simulink model "LF_AC29bus_HVDCdemo_V2_1"  (R2019b)
settings: Solver=FixedStepDiscrete  StartTime=0.0  StopTime=fix(6/Ts)*Ts  FixedStep=Ts  RelTol=1e-3
InitFcn:
  | Ts_avg=150e-6;
  | Ts=50e-6;
  | 
  | %Tc_stab = 1/60/5;
  | %Tc_stab = 2/60;
  | Tc_stab = Ts;
  | 
  | 
  | Ts_avg=150e-6;
  | 
  | Ts=50e-6;
  | 
  | % Rectifier AC side :
  | VLL_nom_R = 735e3; % V
  | Fnom_R = 60;           % Hz
  | 
  | % Inverter AC side :
  | VLL_nom_I = 735e3; % V
  | Fnom_I = 60;           % Hz
  | 
  | % DC :
  | Vdc_nom = 500e3;   % V
  | Idc_nom  = 2000;     % A
undefined symbols (not defined in the file): D1, D11, Delta, test_alpha
libraries: powerlib x223, powerlib_meascontrol x57, simulink x22, sps_avr x7
(part 9 of 10)

== system LF_AC29bus_HVDCdemo_V2_1/HVDC_network_avg/Inverter Control and Protection (Average model)/Inverter Protections/Commutation Failure Prevention Control (CFPREV)/CFPREV ==
  note: Ref. "A Novel Method to Mitigate Commutation Failures in HVDC Systems,"
      | Lidong Zhang, Lars Dofnas ABB Utilities Power System Technology,
      | Proceedings PowerCon 2002, Volume: 1 , 13-17 Oct. 2002,  Page(s): 51-56 vol.1
  note: Silvano Casoria
      | Power System Laboratory, IREQ
      | Hydro-Quebec
  note: Commutation failure Prevention Control (CFPREV)
  note: Fast initialisation
      | for simulation
  Uabc (pu) : Inport
  Enable (Held) : EnablePort  PropagateVarSize=During execution
  AB_LEVEL : Constant  Value=ab_level
  ALPFA_BETA_SUM : Fcn  Expr=sqrt(u[1]^2+u[2]^2)
  ALPFA_BETA_SUM1 : Fcn  Expr=abs(u[3]) * 3
  C : Constant  Value=filt_tc
  C1 : Constant  Value=1/(fn)
  Discrete Shift Register 1 (T_periode) : powerlib_meascontrol/Additional Components/Discrete Shift Register  NSamples=fix(T_periode/Ts)  InitialValue=0  Ts=Ts
      settings: SourceProductName=Simscape Electrical  SourceProductBaseCode=PS
  Discrete Shift Register 2 (T_periode) : powerlib_meascontrol/Additional Components/Discrete Shift Register  NSamples=fix(T_periode/Ts)  InitialValue=0  Ts=Ts
      settings: SourceProductName=Simscape Electrical  SourceProductBaseCode=PS
  First-Order Filter (T=0.03) : powerlib_meascontrol/Filters/First-Order Filter  FilterType=Lowpass  Tc=0.03  Ts=Ts  Initialize=off  Vac_Init=[0, 0, Fnom_I]  Vdc_Init=0  PlotResponse=off  FreqRange="[0,  200,  1]"
      settings: SourceProductName=Simscape Electrical
  Gain : Gain  Gain=ab_gain  SaturateOnIntegerOverflow=on  OutDataTypeStr=Inherit: Same as input  ParamDataTypeStr=Inherit: Same as input
  "Gain  " : Gain  Gain=z_gain  SaturateOnIntegerOverflow=on  OutDataTypeStr=Inherit: Same as input  ParamDataTypeStr=Inherit: Same as input
  Ground : Ground
  Low Pass (IC = filt_ic) : Subsystem  mask(Low Pass Filter With Reset (discrete: Zoh method, Forward Euler)){ic=filt_ic, dt=Ts}
      mask prompts: ic "Initial condition:"; dt "Sample time (s)"
      mask help:
      | The output will be reset to the input value (Time constant = 0)  during the input (2) is True. The Time constant (T) is defined by
      | input (3).
      mask Display:
      | plot(0,0,100,100,[90,80,70,60,50,40,29,20,10],[60,55,52,55,60,65,67,65,60],[89,80,71,60,50,40,30,20,10],[40,35,32,35,40,45,47,45,40],[56,44],[70,50]);
      | disp('\n\nD')
  Max: 1 pu Min = 0 : Saturate  UpperLimit=1.0  LowerLimit=0
  MinMax1 : MinMax  Function=max  SaturateOnIntegerOverflow=on  InputSameDT=on
  MinMax2 : MinMax  Function=max  SaturateOnIntegerOverflow=on  InputSameDT=on
  MinMax3 : MinMax  Function=max  Inputs=2  SaturateOnIntegerOverflow=on  InputSameDT=on
  MinMax4 : MinMax  Function=max  Inputs=2  SaturateOnIntegerOverflow=on  InputSameDT=on
  Relational Operator : RelationalOperator  Operator=>  RndMeth=Nearest
  Relational Operator1 : RelationalOperator  Operator=>  RndMeth=Nearest
  Sum : Sum  Inputs=+-  SaturateOnIntegerOverflow=on
  Switch : Switch  Criteria=u2 > Threshold  SaturateOnIntegerOverflow=on
  Switch1 : Switch  Criteria=u2 > Threshold  SaturateOnIntegerOverflow=on
  Switch2 : Switch  Criteria=u2 > Threshold  SaturateOnIntegerOverflow=on
  T_ss : Step  Time=T_ss  Before=1  After=0  SampleTime=0
  ZERO : Constant  Value=0
  ZERO1 : Constant  Value=0
  Z_LEVEL : Constant  Value=z_level
  abc to Alpha-Beta-Zero : powerlib_meascontrol/Transformations/abc to Alpha-Beta-Zero
      settings: SourceProductName=Simscape Electrical
  AMIN_CFPREV (deg) : Outport
  wires:
  MinMax4/1 -> AMIN_CFPREV (deg)/1
  MinMax3/1 -> First-Order Filter (T=0.03)/1, MinMax4/2
  ALPFA_BETA_SUM/1 -> Low Pass (IC = filt_ic)/1(In), Sum/2
  Sum/1 -> Discrete Shift Register 2 (T_periode)/1, Relational Operator/1
  AB_LEVEL/1 -> Relational Operator/2
  Relational Operator/1 -> Switch/2  "AB_DET"
  Discrete Shift Register 2 (T_periode)/1 -> MinMax1/1
  MinMax1/1 -> Gain/1
  Gain/1 -> Switch/1  "AB_AMIN"
  ZERO/1 -> Switch/3
  ALPFA_BETA_SUM1/1 -> Discrete Shift Register 1 (T_periode)/1, Relational Operator1/1  "Z_DIFF"
  Z_LEVEL/1 -> Relational Operator1/2
  Discrete Shift Register 1 (T_periode)/1 -> MinMax2/1
  MinMax2/1 -> Max: 1 pu Min = 0/1
  Max: 1 pu Min = 0/1 -> "Gain  "/1
  Relational Operator1/1 -> Switch1/2  "Z_DET"
  "Gain  "/1 -> Switch1/1  "Z_AMIN"
  ZERO1/1 -> Switch1/3
  Switch/1 -> MinMax3/1  "AB MIN"
  Switch1/1 -> MinMax3/2  "Z MIN"
  abc to Alpha-Beta-Zero/1 -> ALPFA_BETA_SUM/1, ALPFA_BETA_SUM1/1
  Uabc (pu)/1 -> abc to Alpha-Beta-Zero/1
  Low Pass (IC = filt_ic)/1(Out) -> Sum/1
  Switch2/1 -> Low Pass (IC = filt_ic)/3(T)
  C/1 -> Switch2/3
  T_ss/1 -> Switch2/2
  C1/1 -> Switch2/1
  Ground/1 -> Low Pass (IC = filt_ic)/2(R)
  First-Order Filter (T=0.03)/1 -> MinMax4/1

== system LF_AC29bus_HVDCdemo_V2_1/HVDC_network_avg/Inverter Control and Protection (Average model)/Inverter Protections/Low  AC Voltage Detection (LACVD)/LACVD ==
  note: Low AC Voltage Detection
  Uac (pu) : Inport
  Enable (Held) : EnablePort  PropagateVarSize=During execution
  Off Delay : powerlib_meascontrol/Logic/On Delay  DelayType=Off delay  delay=0.009  ic=0  Ts=Ts
      settings: SourceProductName=Simscape Electrical
  "On Delay 1 " : powerlib_meascontrol/Logic/On Delay  DelayType=On delay  delay=0.001  ic=0  Ts=Ts
      settings: SourceProductName=Simscape Electrical
  On Delay 2 : powerlib_meascontrol/Logic/On Delay  DelayType=On delay  delay=0.014  ic=0  Ts=Ts
      settings: SourceProductName=Simscape Electrical
  REF_1 (pu) : Constant  Value=Ref_1
  Relational Operator1 : RelationalOperator  Operator=<=  RndMeth=Nearest  InputSameDT=on
  Low_AC_Voltage : Outport
  wires:
  REF_1 (pu)/1 -> Relational Operator1/2
  Uac (pu)/1 -> Relational Operator1/1
  "On Delay 1 "/1 -> Off Delay/1
  Off Delay/1 -> On Delay 2/1
  Relational Operator1/1 -> "On Delay 1 "/1
  On Delay 2/1 -> Low_AC_Voltage/1

== system LF_AC29bus_HVDCdemo_V2_1/HVDC_network_avg/Rectifier Average model/HVDC_CONV_AVG/Average Model Computation/Iabc_calc ==
  note: Iabc_calc
  note: Iabc Calculation
  I_dq : Inport
  theta : Inport  Port=2
  Constant : Constant  Value=0
  Mux : Mux  Inputs=[2 1]
  dq0 to abc : powerlib_meascontrol/Transformations/dq0 to abc  Alignment=90 degrees behind phase A axis
      settings: SourceProductName=Simscape Electrical
  rms->peak : Gain  Gain=sqrt(2)
  Iabc : Outport
  wires:
  Mux/1 -> dq0 to abc/1
  dq0 to abc/1 -> Iabc/1
  theta/1 -> dq0 to abc/2
  Constant/1 -> Mux/2
  I_dq/1 -> rms->peak/1
  rms->peak/1 -> Mux/1

== system LF_AC29bus_HVDCdemo_V2_1/HVDC_network_avg/Rectifier Average model/HVDC_CONV_AVG/Average Model Computation/Ud_calc_dyn ==
  note: Derivative
  note: (2 - mu_deg/120) * Lc
  note: dId/dt
  note: Band pass limitation
  note: Output limitation
  note: Ud_calc_dyn
  note: Inductive voltage drop calculation due to current variation
  note: Mean commutation inductance,
      | a function of the commutation interval
  Id : Inport
  mu_deg : Inport  Port=2
  Ud_tmp : Inport  Port=3
  Add : Sum  Inputs=-+
  Difference : Subsystem  mask(Difference){ICPrevInput=0, OutMin=[], OutMax=[], OutDataTypeStr=Inherit: Inherit via internal rule, OutputDataTypeScalingMode=Inherit via internal rule, OutDataType=fixdt(1, 16), OutScaling=2^-10, LockScale=off, RndMeth=Floor, DoSatur=off}
      mask prompts: ICPrevInput "Initial condition for previous input:"; OutMin "Output minimum:"; OutMax "Output maximum:"; OutDataTypeStr "Output data type:"; OutputDataTypeScalingMode "Output data type mode:"; OutDataType "Output data type (e.g. fixdt(1, 16), fixdt('single')):"; OutScaling "Output scaling (Slope, e.g. 2^-9 or [Slope Bias], e.g. [1.25 3]):"; LockScale "Lock output data type setting against changes by the fixed-point tools"; RndMeth "Integer rounding mode:"; DoSatur "Saturate to max or min when overflows occur"
      mask help: Output the current input value minus the previous input value.
      mask init:
      | blkH = gcbh;
      | blkName = getfullname(blkH);
      | 
      | set_param([blkName,'/Diff'], ...
      |     'RndMeth',RndMeth, ...
      | 	'DoSatur',DoSatur);
      mask Callback OutDataTypeStr: fixptdialog(gcbh)
      mask TypeOptions OutputDataTypeScalingMode: double | single | int8 | uint8 | int16 | uint16 | int32 | uint32 | Specify via dialog | Inherit via internal rule | Inherit via back propagation
      mask Callback OutputDataTypeScalingMode: fixptdialog(gcbh)
      mask Callback OutDataType: fixptdialog(gcbh)
      mask TypeOptions RndMeth: Ceiling | Convergent | Floor | Nearest | Round | Simplest | Zero
      mask Display: dpoly([1 -1],[1 0],'z')
  Difference (IC: Ts) : Subsystem  mask(Difference){ICPrevInput=Ts, OutMin=[], OutMax=[], OutDataTypeStr=Inherit: Inherit via internal rule, OutputDataTypeScalingMode=Inherit via internal rule, OutDataType=fixdt(1, 16), OutScaling=2^-10, LockScale=off, RndMeth=Floor, DoSatur=off}
      mask prompts: ICPrevInput "Initial condition for previous input:"; OutMin "Output minimum:"; OutMax "Output maximum:"; OutDataTypeStr "Output data type:"; OutputDataTypeScalingMode "Output data type mode:"; OutDataType "Output data type (e.g. fixdt(1, 16), fixdt('single')):"; OutScaling "Output scaling (Slope, e.g. 2^-9 or [Slope Bias], e.g. [1.25 3]):"; LockScale "Lock output data type setting against changes by the fixed-point tools"; RndMeth "Integer rounding mode:"; DoSatur "Saturate to max or min when overflows occur"
      mask help: Output the current input value minus the previous input value.
      mask init:
      | blkH = gcbh;
      | blkName = getfullname(blkH);
      | 
      | set_param([blkName,'/Diff'], ...
      |     'RndMeth',RndMeth, ...
      | 	'DoSatur',DoSatur);
      mask Callback OutDataTypeStr: fixptdialog(gcbh)
      mask TypeOptions OutputDataTypeScalingMode: double | single | int8 | uint8 | int16 | uint16 | int32 | uint32 | Specify via dialog | Inherit via internal rule | Inherit via back propagation
      mask Callback OutputDataTypeScalingMode: fixptdialog(gcbh)
      mask Callback OutDataType: fixptdialog(gcbh)
      mask TypeOptions RndMeth: Ceiling | Convergent | Floor | Nearest | Round | Simplest | Zero
      mask Display: dpoly([1 -1],[1 0],'z')
  Digital Clock : DigitalClock  SampleTime=Ts
  Divide : Product  Inputs=*/
  Fcn : Fcn  Expr=(2 - u(1)/120)*Lc
  First-Order Filter (T=0.0005) : powerlib_meascontrol/Filters/First-Order Filter  FilterType=Lowpass  Tc=0.0005  Ts=Ts  Initialize=off  Vac_Init=[0, 0, 60]  Vdc_Init=0  PlotResponse=off  FreqRange="[0,  200,  1]"
      settings: SourceProductName=Simscape Electrical
  Max:10*Usec Min:-10*Usec : Saturate  UpperLimit=10*Usec  LowerLimit=-10*Usec
  Product : Product  RndMeth=Zero
  Ud : Outport
  wires:
  Product/1 -> Add/1
  Difference (IC: Ts)/1(Y) -> Divide/2
  Digital Clock/1 -> Difference (IC: Ts)/1(U)
  Id/1 -> Difference/1(U)
  Divide/1 -> First-Order Filter (T=0.0005)/1
  Difference/1(Y) -> Divide/1
  Fcn/1 -> Product/1  "mean_Lc"
  mu_deg/1 -> Fcn/1
  Add/1 -> Max:10*Usec Min:-10*Usec/1
  Ud_tmp/1 -> Add/2
  First-Order Filter (T=0.0005)/1 -> Product/2
  Max:10*Usec Min:-10*Usec/1 -> Ud/1

== system LF_AC29bus_HVDCdemo_V2_1/HVDC_network_avg/Rectifier Average model/HVDC_CONV_AVG/Average Model Computation/Udi0_calc ==
  note: Np/Ns (pu)
  note: Udi0_calc
  note: 3*sqrt(2)/pi * Usec_nom
  note: Udio Calculation
  Uabc : Inport
  Tap_pu : Inport  Port=2
  Avoid zero : Saturate  UpperLimit=inf  LowerLimit=eps
  "Avoid zero " : Saturate  UpperLimit=inf  LowerLimit=eps
  Divide3 : Product  Inputs=*/
  PLL (3ph) : powerlib_meascontrol/PLL/PLL (3ph)  Fmin=0.75 * fn  Par_Init="[0  fn]"  ParK=[60 1400 0]  TcD=Ts  MaxRateChangeFreq=12  FilterCutOffFreq=25  Ts=Ts  AGC=off
      settings: SourceProductName=Simscape Electrical
  Positive-Sequence (PLL-Driven) : powerlib_meascontrol/Measurements/Positive-Sequence (PLL-Driven)  Finit=fn  Fmin=45  InInit=[1, 0]  Ts=Ts
      settings: SourceProductName=Simscape Electrical  SourceProductBaseCode=PS
  Terminator1 : Terminator
  V->pu : Gain  Gain=1/(Uprim/sqrt(1.5))
  V->pu1 : Gain  Gain=2*pi
  delay compensation : Subsystem
  pu->Udio_V : Gain  Gain=(3*sqrt(2)/pi) * Usec
  Udi0 : Outport
  w : Outport  Port=2
  theta : Outport  Port=3
  wires:
  PLL (3ph)/2 -> delay compensation/2(wt_in)
  delay compensation/1(wt_out) -> Positive-Sequence (PLL-Driven)/2, theta/1
  Positive-Sequence (PLL-Driven)/2 -> Terminator1/1
  "Avoid zero "/1 -> Divide3/2
  V->pu1/1 -> delay compensation/1(w), w/1
  PLL (3ph)/1 -> V->pu1/1, Positive-Sequence (PLL-Driven)/1
  Tap_pu/1 -> "Avoid zero "/1
  Divide3/1 -> Udi0/1
  Avoid zero/1 -> Divide3/1
  Uabc/1 -> V->pu/1
  pu->Udio_V/1 -> Avoid zero/1
  V->pu/1 -> PLL (3ph)/1, Positive-Sequence (PLL-Driven)/3
  Positive-Sequence (PLL-Driven)/1 -> pu->Udio_V/1

== system LF_AC29bus_HVDCdemo_V2_1/HVDC_network_avg/Rectifier Control and Protection (Average model)/Rectifier Pole Control (Current)/Current Regulator/PI Regulator with external limits and linrarized Kp (Discrete) ==
  note: PI Regulator With external limits (Linearized Kp) (Discrete)
  Max_i : Inport
  Min_i : Inport  Port=2
  ERR : Inport  Port=3
  Max_pi : Inport  Port=4
  Min_pi : Inport  Port=5
  Alpha_lin : Inport  Port=6
  Max_lin : Inport  Port=7
  Min_lin : Inport  Port=8
  Inv : Inport  Port=9
  Ground : Ground
  Ground1 : Ground
  KI (deg per pu per s) : Gain  Gain=Ki  SaturateOnIntegerOverflow=on  OutDataTypeStr=Inherit: Same as input  ParamDataTypeStr=Inherit: Same as input
  Kp (deg per pu) : Constant  Value=Kp
  Kp Linearisation : Subsystem
  Prod : Product  SaturateOnIntegerOverflow=on  InputSameDT=on  OutDataTypeStr=Inherit: Same as first input
  S16 : Subsystem  mask(Integrator  With  External  Dynamic  Limits (Discrete)){k=1, ic=IC_i, st=pas}
      mask prompts: k "Gain:"; ic "Initial Condition:"; st "Sample time: (s)"
      mask Display: disp('Integrator\nwith\nExternal Limits\nGain & Reset & Hold\n(Discrete)')
  Saturation Dynamic : simulink/Discontinuities/Saturation Dynamic  OutMin=[]  OutMax=[]  OutDataTypeStr=Inherit: Same as second input  OutDataType=fixdt(1, 16)  OutScaling=2^-10  DoSatur=off
  Sum : Sum  SaturateOnIntegerOverflow=on  InputSameDT=on  OutDataTypeStr=Inherit: Same as first input
  Alpha_ord : Outport  InitialOutput=0
  wires:
  Saturation Dynamic/1 -> Alpha_ord/1
  Prod/1 -> Sum/1
  Min_lin/1 -> Kp Linearisation/4(Min_lin)
  Max_lin/1 -> Kp Linearisation/5(Max_lin)
  Inv/1 -> Kp Linearisation/3(Inv)
  ERR/1 -> Prod/2, KI (deg per pu per s)/1
  S16/1(Out) -> Sum/2
  Min_pi/1 -> Saturation Dynamic/3
  Max_pi/1 -> Saturation Dynamic/1
  Sum/1 -> Saturation Dynamic/2
  Min_i/1 -> S16/2(Min)
  Max_i/1 -> S16/1(Max)
  KI (deg per pu per s)/1 -> S16/3(In)
  Kp (deg per pu)/1 -> Kp Linearisation/2(Kp)
  Kp Linearisation/1(Kp_lin) -> Prod/1
  Alpha_lin/1 -> Kp Linearisation/1(Alpha_lin)
  Ground/1 -> S16/4(Reset), S16/5(Hold)
  Ground1/1 -> S16/6(Reset Value)

== system LF_AC29bus_HVDCdemo_V2_1/HVDC_network_avg/Rectifier Control and Protection (Average model)/Rectifier Pole Control (Current)/Gamma Regulator/PI Regulator with external limits and linrarized Kp (Discrete)1 ==
  note: PI Regulator With external limits (Linearized Kp) (Discrete)
  Max_i : Inport
  Min_i : Inport  Port=2
  ERR : Inport  Port=3
  Max_pi : Inport  Port=4
  Min_pi : Inport  Port=5
  Alpha_lin : Inport  Port=6
  Max_lin : Inport  Port=7
  Min_lin : Inport  Port=8
  Inv : Inport  Port=9
  Ground : Ground
  Ground1 : Ground
  KI (deg per pu per s) : Gain  Gain=Ki  SaturateOnIntegerOverflow=on  OutDataTypeStr=Inherit: Same as input  ParamDataTypeStr=Inherit: Same as input
  Kp (deg per pu) : Constant  Value=Kp
  Kp Linearisation : Subsystem
  Prod : Product  SaturateOnIntegerOverflow=on  InputSameDT=on  OutDataTypeStr=Inherit: Same as first input
  S16 : Subsystem  mask(Integrator  With  External  Dynamic  Limits (Discrete)){k=1, ic=IC_i, st=pas}
      mask prompts: k "Gain:"; ic "Initial Condition:"; st "Sample time: (s)"
      mask Display: disp('Integrator\nwith\nExternal Limits\nGain & Reset & Hold\n(Discrete)')
  Saturation Dynamic : simulink/Discontinuities/Saturation Dynamic  OutMin=[]  OutMax=[]  OutDataTypeStr=Inherit: Same as second input  OutDataType=fixdt(1, 16)  OutScaling=2^-10  DoSatur=off
  Sum : Sum  SaturateOnIntegerOverflow=on  InputSameDT=on  OutDataTypeStr=Inherit: Same as first input
  Alpha_ord : Outport  InitialOutput=0
  wires:
  Saturation Dynamic/1 -> Alpha_ord/1
  Prod/1 -> Sum/1
  Min_lin/1 -> Kp Linearisation/4(Min_lin)
  Max_lin/1 -> Kp Linearisation/5(Max_lin)
  Inv/1 -> Kp Linearisation/3(Inv)
  ERR/1 -> Prod/2, KI (deg per pu per s)/1
  S16/1(Out) -> Sum/2
  Min_pi/1 -> Saturation Dynamic/3
  Max_pi/1 -> Saturation Dynamic/1
  Sum/1 -> Saturation Dynamic/2
  Min_i/1 -> S16/2(Min)
  Max_i/1 -> S16/1(Max)
  KI (deg per pu per s)/1 -> S16/3(In)
  Kp (deg per pu)/1 -> Kp Linearisation/2(Kp)
  Kp Linearisation/1(Kp_lin) -> Prod/1
  Alpha_lin/1 -> Kp Linearisation/1(Alpha_lin)
  Ground/1 -> S16/4(Reset), S16/5(Hold)
  Ground1/1 -> S16/6(Reset Value)

== system LF_AC29bus_HVDCdemo_V2_1/HVDC_network_avg/Rectifier Control and Protection (Average model)/Rectifier Pole Control (Current)/Voltage Regulator/PI Regulator with external limits and linrarized Kp (Discrete) ==
  note: PI Regulator With external limits (Linearized Kp) (Discrete)
  Max_i : Inport
  Min_i : Inport  Port=2
  ERR : Inport  Port=3
  Max_pi : Inport  Port=4
  Min_pi : Inport  Port=5
  Alpha_lin : Inport  Port=6
  Max_lin : Inport  Port=7
  Min_lin : Inport  Port=8
  Inv : Inport  Port=9
  Ground : Ground
  Ground1 : Ground
  KI (deg per pu per s) : Gain  Gain=Ki  SaturateOnIntegerOverflow=on  OutDataTypeStr=Inherit: Same as input  ParamDataTypeStr=Inherit: Same as input
  Kp (deg per pu) : Constant  Value=Kp
  Kp Linearisation : Subsystem
  Prod : Product  SaturateOnIntegerOverflow=on  InputSameDT=on  OutDataTypeStr=Inherit: Same as first input
  S16 : Subsystem  mask(Integrator  With  External  Dynamic  Limits (Discrete)){k=1, ic=IC_i, st=pas}
      mask prompts: k "Gain:"; ic "Initial Condition:"; st "Sample time: (s)"
      mask Display: disp('Integrator\nwith\nExternal Limits\nGain & Reset & Hold\n(Discrete)')
  Saturation Dynamic : simulink/Discontinuities/Saturation Dynamic  OutMin=[]  OutMax=[]  OutDataTypeStr=Inherit: Same as second input  OutDataType=fixdt(1, 16)  OutScaling=2^-10  DoSatur=off
  Sum : Sum  SaturateOnIntegerOverflow=on  InputSameDT=on  OutDataTypeStr=Inherit: Same as first input
  Alpha_ord : Outport  InitialOutput=0
  wires:
  Saturation Dynamic/1 -> Alpha_ord/1
  Prod/1 -> Sum/1
  Min_lin/1 -> Kp Linearisation/4(Min_lin)
  Max_lin/1 -> Kp Linearisation/5(Max_lin)
  Inv/1 -> Kp Linearisation/3(Inv)
  ERR/1 -> Prod/2, KI (deg per pu per s)/1
  S16/1(Out) -> Sum/2
  Min_pi/1 -> Saturation Dynamic/3
  Max_pi/1 -> Saturation Dynamic/1
  Sum/1 -> Saturation Dynamic/2
  Min_i/1 -> S16/2(Min)
  Max_i/1 -> S16/1(Max)
  KI (deg per pu per s)/1 -> S16/3(In)
  Kp (deg per pu)/1 -> Kp Linearisation/2(Kp)
  Kp Linearisation/1(Kp_lin) -> Prod/1
  Alpha_lin/1 -> Kp Linearisation/1(Alpha_lin)
  Ground/1 -> S16/4(Reset), S16/5(Hold)
  Ground1/1 -> S16/6(Reset Value)

== system LF_AC29bus_HVDCdemo_V2_1/HVDC_network_avg/Rectifier Control and Protection (Average model)/Rectifier Pole Control (Current)/Voltage dependent Current Order Limiter/Low Pass (IC = 1.0) ==
  note: Low Pass Filter
      | with external Tc & Reset
      | (Zoh methode)
  note: Silvano Casoria
      | Power System Simulation Laboratory
      |  IREQ, Hydro-Quebec
  In : Inport
  R : Inport  Port=2
  T : Inport  Port=3
  Constant : Constant  Value=Ts
  IC= ic : UnitDelay  InitialCondition=ic  SampleTime=dt  HasFrameUpgradeWarning=on
  Math Function : Math  Operator=reciprocal  SaturateOnIntegerOverflow=on
  Product : Product  Inputs=3  SaturateOnIntegerOverflow=on  InputSameDT=on  OutDataTypeStr=Inherit: Same as first input
  Sum : Sum  Inputs=+-  SaturateOnIntegerOverflow=on  InputSameDT=on  OutDataTypeStr=Inherit: Same as first input
  Sum1 : Sum  SaturateOnIntegerOverflow=on  InputSameDT=on  OutDataTypeStr=Inherit: Same as first input
  Switch : Switch  Criteria=u2 > Threshold  SaturateOnIntegerOverflow=on  InputSameDT=on
  Out : Outport
  wires:
  IC= ic/1 -> Sum/2, Sum1/2
  In/1 -> Switch/1, Sum/1
  Sum1/1 -> Out/1, Switch/3
  Switch/1 -> IC= ic/1
  Product/1 -> Sum1/1
  Sum/1 -> Product/2
  Math Function/1 -> Product/1
  T/1 -> Math Function/1
  Constant/1 -> Product/3
  R/1 -> Switch/2

== system LF_AC29bus_HVDCdemo_V2_1/HVDC_network_avg/Rectifier Control and Protection (Average model)/Rectifier Protections/DC Fault Protection (DCPROT)/Enabled Subsystem ==
  note: DC Fault Protection (only in Rectifier)
  VdL (pu) : Inport
  Deblocked : Inport  Port=2  OutDataTypeStr=boolean
  Lock : Inport  Port=3
  Enable (Held) : EnablePort  PropagateVarSize=During execution
  Data Type Conversion : DataTypeConversion  OutDataTypeStr=boolean  SaturateOnIntegerOverflow=on  RndMeth=Zero
  Logical Operator2 : Logic  Inputs=3
  Logical Operator3 : Logic  Operator=NOT
  Logical Operator6 : Logic
  Monostable (T=T2) : powerlib_meascontrol/Logic/Monostable  EdgeDetect=Rising  PulseDuration=T2  ic=0  Ts=Ts
      settings: SourceProductName=Simscape Electrical  SourceProductBaseCode=PS
  ON: -Ref1 (pu) OFF: -(Ref1+0.1) : Relay  OnSwitchValue=-Ref1  OffSwitchValue=-(Ref1 + 0.1)
  "Off Delay 1 " : powerlib_meascontrol/Logic/On Delay  DelayType=Off delay  delay=0.01  ic=0  Ts=Ts
      settings: SourceProductName=Simscape Electrical
  Off Delay 2 : powerlib_meascontrol/Logic/On Delay  DelayType=Off delay  delay=0.16  ic=0  Ts=Ts
      settings: SourceProductName=Simscape Electrical
  On Delay : powerlib_meascontrol/Logic/On Delay  DelayType=On delay  delay=0.2  ic=0  Ts=Ts
      settings: SourceProductName=Simscape Electrical
  On Delay (T=T1) : powerlib_meascontrol/Logic/On Delay  DelayType=On delay  delay=T1  ic=0  Ts=Ts
      settings: SourceProductName=Simscape Electrical
  minus : Gain  Gain=-1  SaturateOnIntegerOverflow=on  OutDataTypeStr=Inherit: Same as input  ParamDataTypeStr=Inherit: Same as input
  voltage sign (pole +) : Gain  Gain=sign  SaturateOnIntegerOverflow=on  OutDataTypeStr=Inherit: Same as input  ParamDataTypeStr=Inherit: Same as input
  Forced_alpha : Outport
  wires:
  minus/1 -> ON: -Ref1 (pu) OFF: -(Ref1+0.1)/1
  Data Type Conversion/1 -> Logical Operator6/1
  On Delay/1 -> Logical Operator6/2
  Logical Operator6/1 -> "Off Delay 1 "/1
  ON: -Ref1 (pu) OFF: -(Ref1+0.1)/1 -> Data Type Conversion/1
  Deblocked/1 -> On Delay/1, Logical Operator2/3
  VdL (pu)/1 -> voltage sign (pole +)/1  "VdL"
  voltage sign (pole +)/1 -> minus/1
  Logical Operator3/1 -> Logical Operator2/2
  Logical Operator2/1 -> On Delay (T=T1)/1
  On Delay (T=T1)/1 -> Monostable (T=T2)/1
  Monostable (T=T2)/1 -> Forced_alpha/1
  "Off Delay 1 "/1 -> Logical Operator2/1
  Lock/1 -> Off Delay 2/1
  Off Delay 2/1 -> Logical Operator3/1

== system LF_AC29bus_HVDCdemo_V2_1/HVDC_network_avg/Rectifier Control and Protection (Average model)/Rectifier Protections/Low  AC Voltage Detection (LACVD)/LACVD ==
  note: Low AC Voltage Detection
  Uac (pu) : Inport
  Enable (Held) : EnablePort  PropagateVarSize=During execution
  Off Delay : powerlib_meascontrol/Logic/On Delay  DelayType=Off delay  delay=0.009  ic=0  Ts=Ts
      settings: SourceProductName=Simscape Electrical
  "On Delay 1 " : powerlib_meascontrol/Logic/On Delay  DelayType=On delay  delay=0.001  ic=0  Ts=Ts
      settings: SourceProductName=Simscape Electrical
  On Delay 2 : powerlib_meascontrol/Logic/On Delay  DelayType=On delay  delay=0.014  ic=0  Ts=Ts
      settings: SourceProductName=Simscape Electrical
  REF_1 (pu) : Constant  Value=Ref_1
  Relational Operator1 : RelationalOperator  Operator=<=  RndMeth=Nearest  InputSameDT=on
  Low_AC_Voltage : Outport
  wires:
  REF_1 (pu)/1 -> Relational Operator1/2
  Uac (pu)/1 -> Relational Operator1/1
  "On Delay 1 "/1 -> Off Delay/1
  Off Delay/1 -> On Delay 2/1
  Relational Operator1/1 -> "On Delay 1 "/1
  On Delay 2/1 -> Low_AC_Voltage/1

== system LF_AC29bus_HVDCdemo_V2_1/HVDC_network_avg/Inverter Average model/HVDC_CONV_AVG/Average Model Computation/Ud_calc_dyn/Difference ==
  note: ( U(k) - U(k-1) )
  note: U(k)
  U : Inport
  Diff : Sum  Description=Add in CPU  Inputs=+-  OutMin=OutMin  OutMax=OutMax  OutDataTypeStr=OutDataTypeStr
  UD : UnitDelay  Description=Store in Global RAM  DisableCoverage=on  InitialCondition=ICPrevInput  SampleTime=-1  HasFrameUpgradeWarning=on
  Y : Outport  OutMin=OutMin  OutMax=OutMax  InitialOutput=0
  wires:
  Diff/1 -> Y/1
  UD/1 -> Diff/2  "U(k-1)"
  U/1 -> Diff/1, UD/1

== system LF_AC29bus_HVDCdemo_V2_1/HVDC_network_avg/Inverter Average model/HVDC_CONV_AVG/Average Model Computation/Ud_calc_dyn/Difference (IC: Ts) ==
  note: U(k)
  note: ( U(k) - U(k-1) )
  U : Inport
  Diff : Sum  Description=Add in CPU  Inputs=+-  OutMin=OutMin  OutMax=OutMax  OutDataTypeStr=OutDataTypeStr
  UD : UnitDelay  Description=Store in Global RAM  DisableCoverage=on  InitialCondition=ICPrevInput  SampleTime=-1  HasFrameUpgradeWarning=on
  Y : Outport  OutMin=OutMin  OutMax=OutMax  InitialOutput=0
  wires:
  U/1 -> UD/1, Diff/1
  UD/1 -> Diff/2  "U(k-1)"
  Diff/1 -> Y/1

== system LF_AC29bus_HVDCdemo_V2_1/HVDC_network_avg/Inverter Average model/HVDC_CONV_AVG/Average Model Computation/Udi0_calc/delay compensation ==
  note: Interface delay compensation
  w : Inport
  wt_in : Inport  Port=2
  Add : Sum
  Delay_time : Gain  Gain=Ts
  wt_out : Outport
  wires:
  w/1 -> Delay_time/1
  Delay_time/1 -> Add/2
  wt_in/1 -> Add/1
  Add/1 -> wt_out/1

== system LF_AC29bus_HVDCdemo_V2_1/HVDC_network_avg/Inverter Control and Protection (Average model)/Inverter Pole Control (Current//Voltage//Gamma)/Current Regulator/PI Regulator with external limits and linrarized Kp (Discrete)/Kp Linearisation ==
  note: Kp Linearization
  Alpha_lin : Inport
  Kp : Inport  Port=2
  Inv : Inport  Port=3
  Min_lin : Inport  Port=4
  Max_lin : Inport  Port=5
  Constant3 : Constant  Value=On_lin
  Data Type Conversion : DataTypeConversion  OutDataTypeStr=boolean  SaturateOnIntegerOverflow=on  RndMeth=Zero
  Logical Operator : Logic  Operator=NOT
  Logical Operator1 : Logic  Operator=NOT
  Math Function : Math  Operator=reciprocal  SaturateOnIntegerOverflow=on
  Prod2 : Product  Inputs=3  SaturateOnIntegerOverflow=on  InputSameDT=on  OutDataTypeStr=Inherit: Same as first input
  Saturation Dynamic : simulink/Discontinuities/Saturation Dynamic  OutMin=[]  OutMax=[]  OutDataTypeStr=Inherit: Same as second input  OutDataType=fixdt(1, 16)  OutScaling=2^-10  DoSatur=off
  Switch : Switch  Criteria=u2 > Threshold  SaturateOnIntegerOverflow=on  InputSameDT=on
  Switch1 : Switch  Criteria=u2 > Threshold  SaturateOnIntegerOverflow=on  InputSameDT=on
  Trigonometric Function : Trigonometry
  Trigonometric Function1 : Trigonometry
  k : Gain  Gain=pi/180  SaturateOnIntegerOverflow=on  OutDataTypeStr=Inherit: Same as input  ParamDataTypeStr=Inherit: Same as input
  k1 : Gain  Gain=pi/180  SaturateOnIntegerOverflow=on  OutDataTypeStr=Inherit: Same as input  ParamDataTypeStr=Inherit: Same as input
  Kp_lin : Outport  InitialOutput=0
  wires:
  Min_lin/1 -> Switch/1, Saturation Dynamic/3
  Max_lin/1 -> Saturation Dynamic/1, Switch/3
  Alpha_lin/1 -> Saturation Dynamic/2
  Math Function/1 -> Prod2/2
  Trigonometric Function1/1 -> Math Function/1
  k/1 -> Trigonometric Function1/1
  Kp/1 -> Switch1/1, Prod2/3
  Inv/1 -> Logical Operator/1
  Logical Operator/1 -> Switch/2
  Trigonometric Function/1 -> Prod2/1
  Saturation Dynamic/1 -> k/1
  k1/1 -> Trigonometric Function/1
  Switch/1 -> k1/1
  Switch1/1 -> Kp_lin/1
  Prod2/1 -> Switch1/3
  Logical Operator1/1 -> Switch1/2  "off"
  Constant3/1 -> Data Type Conversion/1
  Data Type Conversion/1 -> Logical Operator1/1

== system LF_AC29bus_HVDCdemo_V2_1/HVDC_network_avg/Inverter Control and Protection (Average model)/Inverter Pole Control (Current//Voltage//Gamma)/Current Regulator/PI Regulator with external limits and linrarized Kp (Discrete)/S16 ==
  note: INTEGRATOR with External limits & Reset & Hold
  note: Gain * Ts
  Max : Inport
  Min : Inport  Port=2
  In : Inport  Port=3
  Reset : Inport  Port=4
  Hold : Inport  Port=5
  Reset Value : Inport  Port=6
  Gain1 : Gain  Gain=k*st  SaturateOnIntegerOverflow=on  OutDataTypeStr=Inherit: Same as input  ParamDataTypeStr=Inherit: Same as input
  IC = ic : UnitDelay  InitialCondition=ic  SampleTime=st  HasFrameUpgradeWarning=on
  Logical Operator4 : Logic  Operator=OR
  MinMax : MinMax  Inputs=2  SaturateOnIntegerOverflow=on  InputSameDT=on
  MinMax1 : MinMax  Function=max  Inputs=2  SaturateOnIntegerOverflow=on  InputSameDT=on
  Saturation Dynamic : simulink/Discontinuities/Saturation Dynamic  OutMin=[]  OutMax=[]  OutDataTypeStr=Inherit: Same as second input  OutDataType=fixdt(1, 16)  OutScaling=2^-10  DoSatur=off
  Sum : Sum  SaturateOnIntegerOverflow=on  InputSameDT=on  OutDataTypeStr=Inherit: Same as first input
  Switch2 : Switch  Criteria=u2 > Threshold  SaturateOnIntegerOverflow=on  InputSameDT=on
  Switch3 : Switch  Criteria=u2 > Threshold  SaturateOnIntegerOverflow=on  InputSameDT=on
  Switch7 : Switch  Criteria=u2 > Threshold  SaturateOnIntegerOverflow=on  InputSameDT=on
  Out : Outport  InitialOutput=0
  wires:
  Saturation Dynamic/1 -> Out/1, IC = ic/1
  Gain1/1 -> Sum/1
  In/1 -> Gain1/1
  Sum/1 -> Saturation Dynamic/2
  Hold/1 -> Logical Operator4/1
  Reset/1 -> Switch7/2, Logical Operator4/2
  Logical Operator4/1 -> Switch2/2, Switch3/2
  Switch2/1 -> MinMax/1
  Max/1 -> Switch2/3, MinMax/2
  Reset Value/1 -> Switch7/1
  MinMax/1 -> Saturation Dynamic/1
  MinMax1/1 -> Saturation Dynamic/3
  Switch3/1 -> MinMax1/1
  Min/1 -> Switch3/3, MinMax1/2
  IC = ic/1 -> Switch7/3
  Switch7/1 -> Switch3/1, Sum/2, Switch2/1

== system LF_AC29bus_HVDCdemo_V2_1/HVDC_network_avg/Inverter Control and Protection (Average model)/Inverter Pole Control (Current//Voltage//Gamma)/Gamma Regulator/PI Regulator with external limits and linrarized Kp (Discrete)1/Kp Linearisation ==
  note: Kp Linearization
  Alpha_lin : Inport
  Kp : Inport  Port=2
  Inv : Inport  Port=3
  Min_lin : Inport  Port=4
  Max_lin : Inport  Port=5
  Constant3 : Constant  Value=On_lin
  Data Type Conversion : DataTypeConversion  OutDataTypeStr=boolean  SaturateOnIntegerOverflow=on  RndMeth=Zero
  Logical Operator : Logic  Operator=NOT
  Logical Operator1 : Logic  Operator=NOT
  Math Function : Math  Operator=reciprocal  SaturateOnIntegerOverflow=on
  Prod2 : Product  Inputs=3  SaturateOnIntegerOverflow=on  InputSameDT=on  OutDataTypeStr=Inherit: Same as first input
  Saturation Dynamic : simulink/Discontinuities/Saturation Dynamic  OutMin=[]  OutMax=[]  OutDataTypeStr=Inherit: Same as second input  OutDataType=fixdt(1, 16)  OutScaling=2^-10  DoSatur=off
  Switch : Switch  Criteria=u2 > Threshold  SaturateOnIntegerOverflow=on  InputSameDT=on
  Switch1 : Switch  Criteria=u2 > Threshold  SaturateOnIntegerOverflow=on  InputSameDT=on
  Trigonometric Function : Trigonometry
  Trigonometric Function1 : Trigonometry
  k : Gain  Gain=pi/180  SaturateOnIntegerOverflow=on  OutDataTypeStr=Inherit: Same as input  ParamDataTypeStr=Inherit: Same as input
  k1 : Gain  Gain=pi/180  SaturateOnIntegerOverflow=on  OutDataTypeStr=Inherit: Same as input  ParamDataTypeStr=Inherit: Same as input
  Kp_lin : Outport  InitialOutput=0
  wires:
  Min_lin/1 -> Switch/1, Saturation Dynamic/3
  Max_lin/1 -> Saturation Dynamic/1, Switch/3
  Alpha_lin/1 -> Saturation Dynamic/2
  Math Function/1 -> Prod2/2
  Trigonometric Function1/1 -> Math Function/1
  k/1 -> Trigonometric Function1/1
  Kp/1 -> Switch1/1, Prod2/3
  Inv/1 -> Logical Operator/1
  Logical Operator/1 -> Switch/2
  Trigonometric Function/1 -> Prod2/1
  Saturation Dynamic/1 -> k/1
  k1/1 -> Trigonometric Function/1
  Switch/1 -> k1/1
  Switch1/1 -> Kp_lin/1
  Prod2/1 -> Switch1/3
  Logical Operator1/1 -> Switch1/2  "off"
  Constant3/1 -> Data Type Conversion/1
  Data Type Conversion/1 -> Logical Operator1/1

== system LF_AC29bus_HVDCdemo_V2_1/HVDC_network_avg/Inverter Control and Protection (Average model)/Inverter Pole Control (Current//Voltage//Gamma)/Gamma Regulator/PI Regulator with external limits and linrarized Kp (Discrete)1/S16 ==
  note: INTEGRATOR with External limits & Reset & Hold
  note: Gain * Ts
  Max : Inport
  Min : Inport  Port=2
  In : Inport  Port=3
  Reset : Inport  Port=4
  Hold : Inport  Port=5
  Reset Value : Inport  Port=6
  Gain1 : Gain  Gain=k*st  SaturateOnIntegerOverflow=on  OutDataTypeStr=Inherit: Same as input  ParamDataTypeStr=Inherit: Same as input
  IC = ic : UnitDelay  InitialCondition=ic  SampleTime=st  HasFrameUpgradeWarning=on
  Logical Operator4 : Logic  Operator=OR
  MinMax : MinMax  Inputs=2  SaturateOnIntegerOverflow=on  InputSameDT=on
  MinMax1 : MinMax  Function=max  Inputs=2  SaturateOnIntegerOverflow=on  InputSameDT=on
  Saturation Dynamic : simulink/Discontinuities/Saturation Dynamic  OutMin=[]  OutMax=[]  OutDataTypeStr=Inherit: Same as second input  OutDataType=fixdt(1, 16)  OutScaling=2^-10  DoSatur=off
  Sum : Sum  SaturateOnIntegerOverflow=on  InputSameDT=on  OutDataTypeStr=Inherit: Same as first input
  Switch2 : Switch  Criteria=u2 > Threshold  SaturateOnIntegerOverflow=on  InputSameDT=on
  Switch3 : Switch  Criteria=u2 > Threshold  SaturateOnIntegerOverflow=on  InputSameDT=on
  Switch7 : Switch  Criteria=u2 > Threshold  SaturateOnIntegerOverflow=on  InputSameDT=on
  Out : Outport  InitialOutput=0
  wires:
  Saturation Dynamic/1 -> Out/1, IC = ic/1
  Gain1/1 -> Sum/1
  In/1 -> Gain1/1
  Sum/1 -> Saturation Dynamic/2
  Hold/1 -> Logical Operator4/1
  Reset/1 -> Switch7/2, Logical Operator4/2
  Logical Operator4/1 -> Switch2/2, Switch3/2
  Switch2/1 -> MinMax/1
  Max/1 -> Switch2/3, MinMax/2
  Reset Value/1 -> Switch7/1
  MinMax/1 -> Saturation Dynamic/1
  MinMax1/1 -> Saturation Dynamic/3
  Switch3/1 -> MinMax1/1
  Min/1 -> Switch3/3, MinMax1/2
  IC = ic/1 -> Switch7/3
  Switch7/1 -> Switch3/1, Sum/2, Switch2/1

== system LF_AC29bus_HVDCdemo_V2_1/HVDC_network_avg/Inverter Control and Protection (Average model)/Inverter Pole Control (Current//Voltage//Gamma)/Voltage Regulator/PI Regulator with external limits and linrarized Kp (Discrete)/Kp Linearisation ==
  note: Kp Linearization
  Alpha_lin : Inport
  Kp : Inport  Port=2
  Inv : Inport  Port=3
  Min_lin : Inport  Port=4
  Max_lin : Inport  Port=5
  Constant3 : Constant  Value=On_lin
  Data Type Conversion : DataTypeConversion  OutDataTypeStr=boolean  SaturateOnIntegerOverflow=on  RndMeth=Zero
  Logical Operator : Logic  Operator=NOT
  Logical Operator1 : Logic  Operator=NOT
  Math Function : Math  Operator=reciprocal  SaturateOnIntegerOverflow=on
  Prod2 : Product  Inputs=3  SaturateOnIntegerOverflow=on  InputSameDT=on  OutDataTypeStr=Inherit: Same as first input
  Saturation Dynamic : simulink/Discontinuities/Saturation Dynamic  OutMin=[]  OutMax=[]  OutDataTypeStr=Inherit: Same as second input  OutDataType=fixdt(1, 16)  OutScaling=2^-10  DoSatur=off
  Switch : Switch  Criteria=u2 > Threshold  SaturateOnIntegerOverflow=on  InputSameDT=on
  Switch1 : Switch  Criteria=u2 > Threshold  SaturateOnIntegerOverflow=on  InputSameDT=on
  Trigonometric Function : Trigonometry
  Trigonometric Function1 : Trigonometry
  k : Gain  Gain=pi/180  SaturateOnIntegerOverflow=on  OutDataTypeStr=Inherit: Same as input  ParamDataTypeStr=Inherit: Same as input
  k1 : Gain  Gain=pi/180  SaturateOnIntegerOverflow=on  OutDataTypeStr=Inherit: Same as input  ParamDataTypeStr=Inherit: Same as input
  Kp_lin : Outport  InitialOutput=0
  wires:
  Min_lin/1 -> Switch/1, Saturation Dynamic/3
  Max_lin/1 -> Saturation Dynamic/1, Switch/3
  Alpha_lin/1 -> Saturation Dynamic/2
  Math Function/1 -> Prod2/2
  Trigonometric Function1/1 -> Math Function/1
  k/1 -> Trigonometric Function1/1
  Kp/1 -> Switch1/1, Prod2/3
  Inv/1 -> Logical Operator/1
  Logical Operator/1 -> Switch/2
  Trigonometric Function/1 -> Prod2/1
  Saturation Dynamic/1 -> k/1
  k1/1 -> Trigonometric Function/1
  Switch/1 -> k1/1
  Switch1/1 -> Kp_lin/1
  Prod2/1 -> Switch1/3
  Logical Operator1/1 -> Switch1/2  "off"
  Constant3/1 -> Data Type Conversion/1
  Data Type Conversion/1 -> Logical Operator1/1

== system LF_AC29bus_HVDCdemo_V2_1/HVDC_network_avg/Inverter Control and Protection (Average model)/Inverter Pole Control (Current//Voltage//Gamma)/Voltage Regulator/PI Regulator with external limits and linrarized Kp (Discrete)/S16 ==
  note: INTEGRATOR with External limits & Reset & Hold
  note: Gain * Ts
  Max : Inport
  Min : Inport  Port=2
  In : Inport  Port=3
  Reset : Inport  Port=4
  Hold : Inport  Port=5
  Reset Value : Inport  Port=6
  Gain1 : Gain  Gain=k*st  SaturateOnIntegerOverflow=on  OutDataTypeStr=Inherit: Same as input  ParamDataTypeStr=Inherit: Same as input
  IC = ic : UnitDelay  InitialCondition=ic  SampleTime=st  HasFrameUpgradeWarning=on
  Logical Operator4 : Logic  Operator=OR
  MinMax : MinMax  Inputs=2  SaturateOnIntegerOverflow=on  InputSameDT=on
  MinMax1 : MinMax  Function=max  Inputs=2  SaturateOnIntegerOverflow=on  InputSameDT=on
  Saturation Dynamic : simulink/Discontinuities/Saturation Dynamic  OutMin=[]  OutMax=[]  OutDataTypeStr=Inherit: Same as second input  OutDataType=fixdt(1, 16)  OutScaling=2^-10  DoSatur=off
  Sum : Sum  SaturateOnIntegerOverflow=on  InputSameDT=on  OutDataTypeStr=Inherit: Same as first input
  Switch2 : Switch  Criteria=u2 > Threshold  SaturateOnIntegerOverflow=on  InputSameDT=on
  Switch3 : Switch  Criteria=u2 > Threshold  SaturateOnIntegerOverflow=on  InputSameDT=on
  Switch7 : Switch  Criteria=u2 > Threshold  SaturateOnIntegerOverflow=on  InputSameDT=on
  Out : Outport  InitialOutput=0
  wires:
  Saturation Dynamic/1 -> Out/1, IC = ic/1
  Gain1/1 -> Sum/1
  In/1 -> Gain1/1
  Sum/1 -> Saturation Dynamic/2
  Hold/1 -> Logical Operator4/1
  Reset/1 -> Switch7/2, Logical Operator4/2
  Logical Operator4/1 -> Switch2/2, Switch3/2
  Switch2/1 -> MinMax/1
  Max/1 -> Switch2/3, MinMax/2
  Reset Value/1 -> Switch7/1
  MinMax/1 -> Saturation Dynamic/1
  MinMax1/1 -> Saturation Dynamic/3
  Switch3/1 -> MinMax1/1
  Min/1 -> Switch3/3, MinMax1/2
  IC = ic/1 -> Switch7/3
  Switch7/1 -> Switch3/1, Sum/2, Switch2/1

== system LF_AC29bus_HVDCdemo_V2_1/HVDC_network_avg/Inverter Control and Protection (Average model)/Inverter Protections/Commutation Failure Prevention Control (CFPREV)/CFPREV/Low Pass (IC = filt_ic) ==
  note: Low Pass Filter
      | with external Tc & Reset
      | (Zoh methode)
  note: Silvano Casoria
      | Power System Simulation Laboratory
      |  IREQ, Hydro-Quebec
  In : Inport
  R : Inport  Port=2
  T : Inport  Port=3
  Constant : Constant  Value=Ts
  IC= ic : UnitDelay  InitialCondition=ic  SampleTime=dt  HasFrameUpgradeWarning=on
  Math Function : Math  Operator=reciprocal  SaturateOnIntegerOverflow=on
  Product : Product  Inputs=3  SaturateOnIntegerOverflow=on  InputSameDT=on  OutDataTypeStr=Inherit: Same as first input
  Sum : Sum  Inputs=+-  SaturateOnIntegerOverflow=on  InputSameDT=on  OutDataTypeStr=Inherit: Same as first input
  Sum1 : Sum  SaturateOnIntegerOverflow=on  InputSameDT=on  OutDataTypeStr=Inherit: Same as first input
  Switch : Switch  Criteria=u2 > Threshold  SaturateOnIntegerOverflow=on  InputSameDT=on
  Out : Outport
  wires:
  IC= ic/1 -> Sum/2, Sum1/2
  In/1 -> Switch/1, Sum/1
  Sum1/1 -> Out/1, Switch/3
  Switch/1 -> IC= ic/1
  Product/1 -> Sum1/1
  Sum/1 -> Product/2
  Math Function/1 -> Product/1
  T/1 -> Math Function/1
  Constant/1 -> Product/3
  R/1 -> Switch/2

== system LF_AC29bus_HVDCdemo_V2_1/HVDC_network_avg/Rectifier Average model/HVDC_CONV_AVG/Average Model Computation/Ud_calc_dyn/Difference ==
  note: ( U(k) - U(k-1) )
  note: U(k)
  U : Inport
  Diff : Sum  Description=Add in CPU  Inputs=+-  OutMin=OutMin  OutMax=OutMax  OutDataTypeStr=OutDataTypeStr
  UD : UnitDelay  Description=Store in Global RAM  DisableCoverage=on  InitialCondition=ICPrevInput  SampleTime=-1  HasFrameUpgradeWarning=on
  Y : Outport  OutMin=OutMin  OutMax=OutMax  InitialOutput=0
  wires:
  Diff/1 -> Y/1
  UD/1 -> Diff/2  "U(k-1)"
  U/1 -> Diff/1, UD/1

== system LF_AC29bus_HVDCdemo_V2_1/HVDC_network_avg/Rectifier Average model/HVDC_CONV_AVG/Average Model Computation/Ud_calc_dyn/Difference (IC: Ts) ==
  note: U(k)
  note: ( U(k) - U(k-1) )
  U : Inport
  Diff : Sum  Description=Add in CPU  Inputs=+-  OutMin=OutMin  OutMax=OutMax  OutDataTypeStr=OutDataTypeStr
  UD : UnitDelay  Description=Store in Global RAM  DisableCoverage=on  InitialCondition=ICPrevInput  SampleTime=-1  HasFrameUpgradeWarning=on
  Y : Outport  OutMin=OutMin  OutMax=OutMax  InitialOutput=0
  wires:
  U/1 -> UD/1, Diff/1
  UD/1 -> Diff/2  "U(k-1)"
  Diff/1 -> Y/1

== system LF_AC29bus_HVDCdemo_V2_1/HVDC_network_avg/Rectifier Average model/HVDC_CONV_AVG/Average Model Computation/Udi0_calc/delay compensation ==
  note: Interface delay compensation
  w : Inport
  wt_in : Inport  Port=2
  Add : Sum
  Delay_time : Gain  Gain=Ts
  wt_out : Outport
  wires:
  w/1 -> Delay_time/1
  Delay_time/1 -> Add/2
  wt_in/1 -> Add/1
  Add/1 -> wt_out/1

== system LF_AC29bus_HVDCdemo_V2_1/HVDC_network_avg/Rectifier Control and Protection (Average model)/Rectifier Pole Control (Current)/Current Regulator/PI Regulator with external limits and linrarized Kp (Discrete)/Kp Linearisation ==
  note: Kp Linearization
  Alpha_lin : Inport
  Kp : Inport  Port=2
  Inv : Inport  Port=3
  Min_lin : Inport  Port=4
  Max_lin : Inport  Port=5
  Constant3 : Constant  Value=On_lin
  Data Type Conversion : DataTypeConversion  OutDataTypeStr=boolean  SaturateOnIntegerOverflow=on  RndMeth=Zero
  Logical Operator : Logic  Operator=NOT
  Logical Operator1 : Logic  Operator=NOT
  Math Function : Math  Operator=reciprocal  SaturateOnIntegerOverflow=on
  Prod2 : Product  Inputs=3  SaturateOnIntegerOverflow=on  InputSameDT=on  OutDataTypeStr=Inherit: Same as first input
  Saturation Dynamic : simulink/Discontinuities/Saturation Dynamic  OutMin=[]  OutMax=[]  OutDataTypeStr=Inherit: Same as second input  OutDataType=fixdt(1, 16)  OutScaling=2^-10  DoSatur=off
  Switch : Switch  Criteria=u2 > Threshold  SaturateOnIntegerOverflow=on  InputSameDT=on
  Switch1 : Switch  Criteria=u2 > Threshold  SaturateOnIntegerOverflow=on  InputSameDT=on
  Trigonometric Function : Trigonometry
  Trigonometric Function1 : Trigonometry
  k : Gain  Gain=pi/180  SaturateOnIntegerOverflow=on  OutDataTypeStr=Inherit: Same as input  ParamDataTypeStr=Inherit: Same as input
  k1 : Gain  Gain=pi/180  SaturateOnIntegerOverflow=on  OutDataTypeStr=Inherit: Same as input  ParamDataTypeStr=Inherit: Same as input
  Kp_lin : Outport  InitialOutput=0
  wires:
  Min_lin/1 -> Switch/1, Saturation Dynamic/3
  Max_lin/1 -> Saturation Dynamic/1, Switch/3
  Alpha_lin/1 -> Saturation Dynamic/2
  Math Function/1 -> Prod2/2
  Trigonometric Function1/1 -> Math Function/1
  k/1 -> Trigonometric Function1/1
  Kp/1 -> Switch1/1, Prod2/3
  Inv/1 -> Logical Operator/1
  Logical Operator/1 -> Switch/2
  Trigonometric Function/1 -> Prod2/1
  Saturation Dynamic/1 -> k/1
  k1/1 -> Trigonometric Function/1
  Switch/1 -> k1/1
  Switch1/1 -> Kp_lin/1
  Prod2/1 -> Switch1/3
  Logical Operator1/1 -> Switch1/2  "off"
  Constant3/1 -> Data Type Conversion/1
  Data Type Conversion/1 -> Logical Operator1/1

== system LF_AC29bus_HVDCdemo_V2_1/HVDC_network_avg/Rectifier Control and Protection (Average model)/Rectifier Pole Control (Current)/Current Regulator/PI Regulator with external limits and linrarized Kp (Discrete)/S16 ==
  note: INTEGRATOR with External limits & Reset & Hold
  note: Gain * Ts
  Max : Inport
  Min : Inport  Port=2
  In : Inport  Port=3
  Reset : Inport  Port=4
  Hold : Inport  Port=5
  Reset Value : Inport  Port=6
  Gain1 : Gain  Gain=k*st  SaturateOnIntegerOverflow=on  OutDataTypeStr=Inherit: Same as input  ParamDataTypeStr=Inherit: Same as input
  IC = ic : UnitDelay  InitialCondition=ic  SampleTime=st  HasFrameUpgradeWarning=on
  Logical Operator4 : Logic  Operator=OR
  MinMax : MinMax  Inputs=2  SaturateOnIntegerOverflow=on  InputSameDT=on
  MinMax1 : MinMax  Function=max  Inputs=2  SaturateOnIntegerOverflow=on  InputSameDT=on
  Saturation Dynamic : simulink/Discontinuities/Saturation Dynamic  OutMin=[]  OutMax=[]  OutDataTypeStr=Inherit: Same as second input  OutDataType=fixdt(1, 16)  OutScaling=2^-10  DoSatur=off
  Sum : Sum  SaturateOnIntegerOverflow=on  InputSameDT=on  OutDataTypeStr=Inherit: Same as first input
  Switch2 : Switch  Criteria=u2 > Threshold  SaturateOnIntegerOverflow=on  InputSameDT=on
  Switch3 : Switch  Criteria=u2 > Threshold  SaturateOnIntegerOverflow=on  InputSameDT=on
  Switch7 : Switch  Criteria=u2 > Threshold  SaturateOnIntegerOverflow=on  InputSameDT=on
  Out : Outport  InitialOutput=0
  wires:
  Saturation Dynamic/1 -> Out/1, IC = ic/1
  Gain1/1 -> Sum/1
  In/1 -> Gain1/1
  Sum/1 -> Saturation Dynamic/2
  Hold/1 -> Logical Operator4/1
  Reset/1 -> Switch7/2, Logical Operator4/2
  Logical Operator4/1 -> Switch2/2, Switch3/2
  Switch2/1 -> MinMax/1
  Max/1 -> Switch2/3, MinMax/2
  Reset Value/1 -> Switch7/1
  MinMax/1 -> Saturation Dynamic/1
  MinMax1/1 -> Saturation Dynamic/3
  Switch3/1 -> MinMax1/1
  Min/1 -> Switch3/3, MinMax1/2
  IC = ic/1 -> Switch7/3
  Switch7/1 -> Switch3/1, Sum/2, Switch2/1

== system LF_AC29bus_HVDCdemo_V2_1/HVDC_network_avg/Rectifier Control and Protection (Average model)/Rectifier Pole Control (Current)/Gamma Regulator/PI Regulator with external limits and linrarized Kp (Discrete)1/Kp Linearisation ==
  note: Kp Linearization
  Alpha_lin : Inport
  Kp : Inport  Port=2
  Inv : Inport  Port=3
  Min_lin : Inport  Port=4
  Max_lin : Inport  Port=5
  Constant3 : Constant  Value=On_lin
  Data Type Conversion : DataTypeConversion  OutDataTypeStr=boolean  SaturateOnIntegerOverflow=on  RndMeth=Zero
  Logical Operator : Logic  Operator=NOT
  Logical Operator1 : Logic  Operator=NOT
  Math Function : Math  Operator=reciprocal  SaturateOnIntegerOverflow=on
  Prod2 : Product  Inputs=3  SaturateOnIntegerOverflow=on  InputSameDT=on  OutDataTypeStr=Inherit: Same as first input
  Saturation Dynamic : simulink/Discontinuities/Saturation Dynamic  OutMin=[]  OutMax=[]  OutDataTypeStr=Inherit: Same as second input  OutDataType=fixdt(1, 16)  OutScaling=2^-10  DoSatur=off
  Switch : Switch  Criteria=u2 > Threshold  SaturateOnIntegerOverflow=on  InputSameDT=on
  Switch1 : Switch  Criteria=u2 > Threshold  SaturateOnIntegerOverflow=on  InputSameDT=on
  Trigonometric Function : Trigonometry
  Trigonometric Function1 : Trigonometry
  k : Gain  Gain=pi/180  SaturateOnIntegerOverflow=on  OutDataTypeStr=Inherit: Same as input  ParamDataTypeStr=Inherit: Same as input
  k1 : Gain  Gain=pi/180  SaturateOnIntegerOverflow=on  OutDataTypeStr=Inherit: Same as input  ParamDataTypeStr=Inherit: Same as input
  Kp_lin : Outport  InitialOutput=0
  wires:
  Min_lin/1 -> Switch/1, Saturation Dynamic/3
  Max_lin/1 -> Saturation Dynamic/1, Switch/3
  Alpha_lin/1 -> Saturation Dynamic/2
  Math Function/1 -> Prod2/2
  Trigonometric Function1/1 -> Math Function/1
  k/1 -> Trigonometric Function1/1
  Kp/1 -> Switch1/1, Prod2/3
  Inv/1 -> Logical Operator/1
  Logical Operator/1 -> Switch/2
  Trigonometric Function/1 -> Prod2/1
  Saturation Dynamic/1 -> k/1
  k1/1 -> Trigonometric Function/1
  Switch/1 -> k1/1
  Switch1/1 -> Kp_lin/1
  Prod2/1 -> Switch1/3
  Logical Operator1/1 -> Switch1/2  "off"
  Constant3/1 -> Data Type Conversion/1
  Data Type Conversion/1 -> Logical Operator1/1
